simulink model "c28x_ccp_ert"  (R2021b)
settings: Solver=FixedStepDiscrete  StartTime=0.0  StopTime=inf  FixedStep=0.01  RelTol=1e-3  EnableMultiTasking=on
PreLoadFcn:
  | RTWConfigurationCB('preloadfcn', bdroot);c2000_ccp_data;
values from neighbouring files (symbols this model uses):
  STEP_PARAM = tic2000demospkg.Parameter    [c2000_ccp_data.m]
libraries: c280xlib x1, demo_controls x1
settings Model: SimulationMode=external  ExtModeEnableFloating=off  Creator=The MathWorks, Inc.  LastModifiedBy=The MathWorks, Inc.
settings SolverCC: AlgebraicLoopSolver=TrustRegion
settings DataIOCC: LimitDataPoints=on  SaveFormat=Array  SaveOutput=off  SaveTime=off  ReturnWorkspaceOutputs=off
settings OptimizationCC: DefaultParameterBehavior=Inlined  ExpressionDepthLimit=2147483647  InitFltsAndDblsToZero=on  LifeSpan=inf  MaxStackSize=64  EfficientTunableParamExpr=on
settings DebuggingCC: UnderspecifiedInitializationDetection=Classic  MergeDetectMultiDrivingBlocksExec=none  CheckExecutionContextPreStartOutputMsg=on  SignalResolutionControl=TryResolveAllWithWarning  SolverPrmCheckMsg=warning  MultiTaskDSMMsg=warning  MultiTaskCondExecSysMsg=none  SigSpecEnsureSampleTimeMsg=none  FcnCallInpInsideContextMsg=warning  AllowSymbolicDim=off  StateNameClashWarn=warning  SFUnexpectedBacktrackingDiag=warning  SFNoUnconditionalDefaultTransitionDiag=warning  SFExecutionAtInitializationDiag=none  SFMachineParentedDataDiag=warning  ArithmeticOperatorsInVariantConditions=warning
settings HardwareCC: ProdBitPerChar=16  ProdBitPerInt=16  ProdBitPerPointer=32  ProdLargestAtomicInteger=Integer  ProdLargestAtomicFloat=None  ProdWordSize=16  ProdHWDeviceType=Texas Instruments->C2000  TargetBitPerChar=16  TargetBitPerInt=16  TargetBitPerPointer=16  TargetLargestAtomicInteger=Integer  TargetIntDivRoundTo=Zero  TargetEndianess=LittleEndian  TargetWordSize=16  TargetHWDeviceType=Texas Instruments->C2000  ProdEqTarget=off
settings ModelReferenceCC: PropagateSignalLabelsOutOfModel=off
settings SFSimCC: SimUseLocalCustomCode=off  SimParseCustomCode=off  MATLABDynamicMemAlloc=off  CustomCodeUndefinedFunction=UseInterfaceOnly
settings RTWCC: Description=Embedded Coder  SystemTargetFile=ert.tlc  HardwareBoard=TI Delfino F2833x  TemplateMakefile=ert_default_tmf  PostCodeGenCommand=; codertarget.postCodeGenHookCommand(h)  RTWUseLocalCustomCode=off  Toolchain=Texas Instruments Code Composer Studio (C2000)
settings CodeAppCC: ForceParamTrailComments=on  IgnoreCustomStorageClasses=off  CustomSymbolStrType=$N$R$M  StateflowObjectComments=on  InternalIdentifier=Classic
settings ERTTargetCC: MultiwordLength=2048  ParMdlRefBuildCompliant=off  CompOptLevelCompliant=off  CPPClassGenCompliant=off  ExtModeStaticAllocSize=2048  ExtModeMexFile=TIC2000ExternalModeOpen  ExtModeIntrfLevel=Level2 - Open  InlinedParameterPlacement=NonHierarchical  ConvertIfToSwitch=off  SuppressUnreachableDefaultCases=off
settings ConfigComp: CovSaveCumulativeToWorkspaceVar=on  CovSaveSingleToWorkspaceVar=on  CovExternalEMLEnable=off  CovSFcnEnable=off

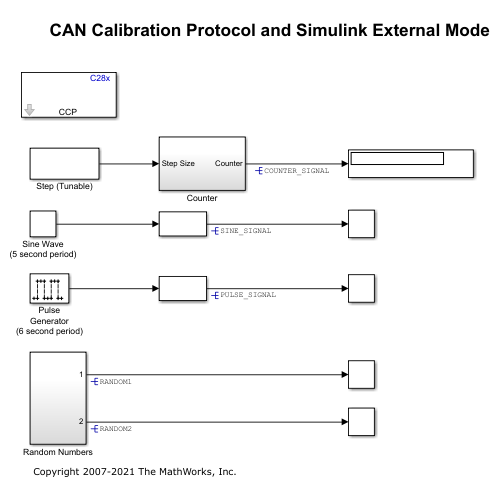
[thumbnail: Simulink's stored preview of the top-level diagram]
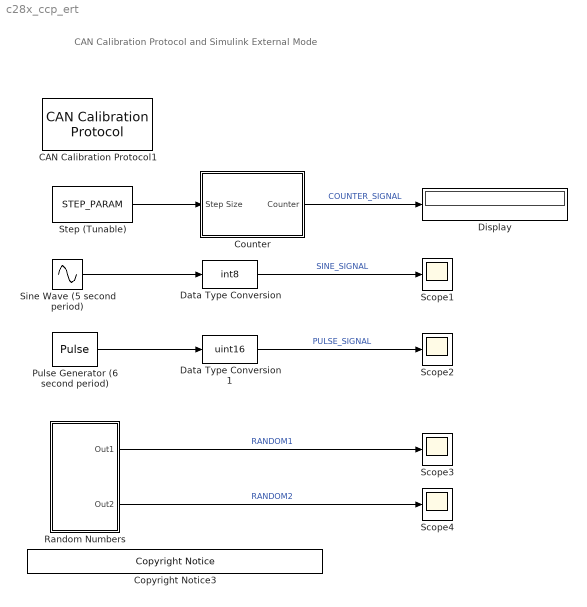
== system c28x_ccp_ert ==
  note: CAN Calibration Protocol and Simulink External Mode
  CAN Calibration Protocol1 : c280xlib/CAN Calibration Protocol  CCP_STATION_ID=hex2dec('1')  module=eCAN_A  ccp_cro_id=hex2dec('6FA')  ccp_cro_message_type=Standard (11-bit identifier)  ccp_return_id=hex2dec('6FB')  ccp_return_message_type=Standard (11-bit identifier)  TOTAL_NUM_ODTS=25  cro_sample_time=0.01
      settings: SourceProductBaseCode=TIC2000
  Copyright Notice3 : demo_controls/Copyright Notice  year=2007  prod=tic2000
      settings: SourceProductBaseCode=ME
  Counter : Subsystem
  Data Type Conversion : DataTypeConversion  OutDataTypeStr=int8  RndMeth=Zero
  Data Type Conversion1 : DataTypeConversion  OutDataTypeStr=uint16
  Display : Display
  Pulse Generator (6 second period) : DiscretePulseGenerator  Amplitude=60000  Period=12  PulseWidth=4  SampleTime=0.5
  Random Numbers : Subsystem
  Scope{1..4} (4 alike) : Scope
  Sine Wave (5 second period) : Sin  SineType=Sample based  Amplitude=125  Samples=50  SampleTime=0.1
  Step (Tunable) : Constant  Value=STEP_PARAM
  wires:
  Step (Tunable)/1 -> Counter/1(Step Size)
  Counter/1(Counter) -> Display/1  "COUNTER_SIGNAL"
  Sine Wave (5 second period)/1 -> Data Type Conversion/1
  Data Type Conversion/1 -> Scope1/1  "SINE_SIGNAL"
  Pulse Generator (6 second period)/1 -> Data Type Conversion1/1
  Data Type Conversion1/1 -> Scope2/1  "PULSE_SIGNAL"
  Random Numbers/2(Out2) -> Scope4/1  "RANDOM2"
  Random Numbers/1(Out1) -> Scope3/1  "RANDOM1"

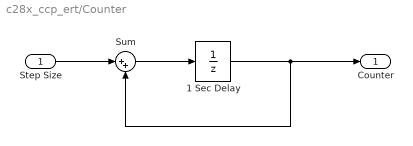
== system c28x_ccp_ert/Counter ==
  Step Size : Inport
  1 Sec Delay : UnitDelay  HasFrameUpgradeWarning=on
  Sum : Sum  Inputs=|++  InputSameDT=on  SaturateOnIntegerOverflow=on  OutDataTypeStr=Inherit: Same as first input
  Counter : Outport
  wires:
  Sum/1 -> 1 Sec Delay/1
  1 Sec Delay/1 -> Sum/2, Counter/1
  Step Size/1 -> Sum/1

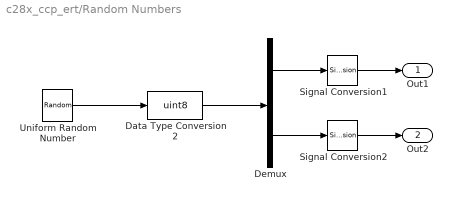
== system c28x_ccp_ert/Random Numbers ==
  Data Type Conversion2 : DataTypeConversion  OutDataTypeStr=uint8
  Demux : Demux  Outputs=2
  Signal Conversion1 : SignalConversion  ConversionOutput=Contiguous copy  OverrideOpt=off
  Signal Conversion2 : SignalConversion  ConversionOutput=Contiguous copy  OverrideOpt=off
  Uniform Random Number : UniformRandomNumber  Minimum=0  Maximum=10  Seed=[1 2]  SampleTime=1
  Out1 : Outport
  Out2 : Outport  Port=2
  wires:
  Uniform Random Number/1 -> Data Type Conversion2/1
  Data Type Conversion2/1 -> Demux/1
  Demux/1 -> Signal Conversion1/1
  Demux/2 -> Signal Conversion2/1
  Signal Conversion1/1 -> Out1/1
  Signal Conversion2/1 -> Out2/1
